simulink model "segway_ctrl_dt"  (R2020a)
settings: Solver=daessc  StartTime=0.0  StopTime=simlength  MaxStep=ts  RelTol=1e-3
values from neighbouring files (symbols this model uses):
  Ad = eye(4) + A*ts    [init_segway_ctrl.m]
  Aled = eye(5) + Ale*ts    [init_segway_ctrl.m]
  Bd = B*ts    [init_segway_ctrl.m]
  Bled = Ble*ts    [init_segway_ctrl.m]
  C = [1 0 0 0; 0 0 1 0]    [init_segway_ctrl.m]
  Cle = [1 0 0 0 0; 0 0 1 0 0]    [init_segway_ctrl.m]
  g = 9.8    [init_segway_ctrl.m]
  K1ed = (K1_hat+[0 0 0 0 1])/([Ad-eye(4) Bd; C1*Ad C1*Bd])    [init_segway_ctrl.m]
  K2ed = (K2_hat+[0 0 0 0 1])/([Ad-eye(4) Bd; C1*Ad C1*Bd])    [init_segway_ctrl.m]
  Ld = (place(Ad',C',poles_obsd))'    [init_segway_ctrl.m]
  Lled = (place(Aled',Cle',poles_obsd_le))'    [init_segway_ctrl.m]
  omega_1_ref = vref/r1    (= 28.5714285714)    [init_segway_ctrl.m]
  simlength = 20    [init_segway_ctrl.m]
  ts = 1e-3    (= 0.001)    [init_segway_ctrl.m]
libraries: nesl_utility x21, fl_lib x6, simulink x3, segway_lib x3
settings Model: SimulationMode=accelerator  Creator=dbagn  LastModifiedBy=dbagn
settings DataIOCC: ReturnWorkspaceOutputs=off

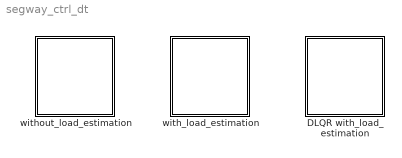
== system segway_ctrl_dt ==
  DLQR with_load_estimation : Subsystem
  with_load_estimation : Subsystem
  without_load_estimation : Subsystem

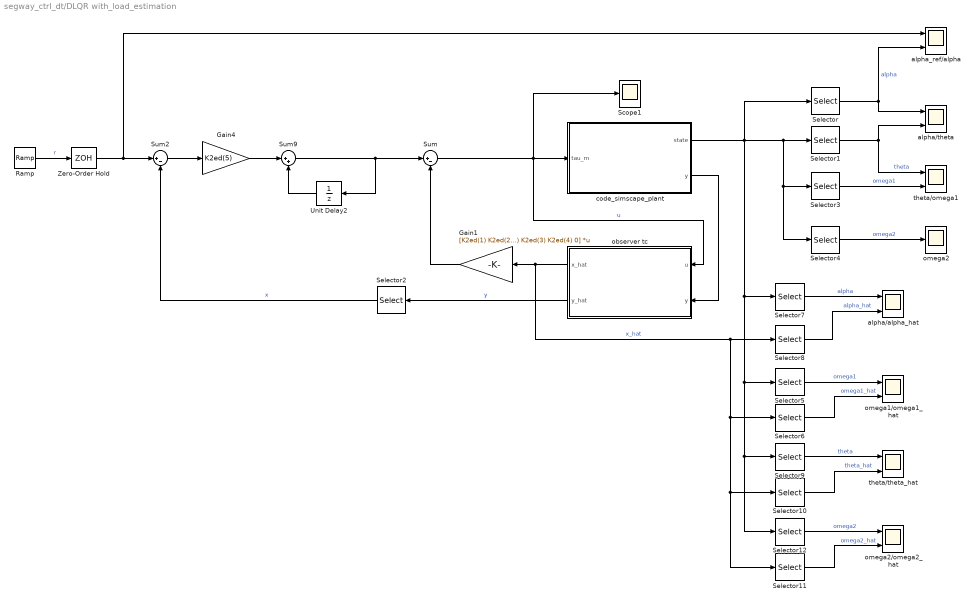
== system segway_ctrl_dt/DLQR with_load_estimation ==
  Gain1 : Gain  Gain=[K2ed(1) K2ed(2) K2ed(3) K2ed(4) 0]  Multiplication=Matrix(K*u)
  Gain4 : Gain  Gain=K2ed(5)
  Ramp : simulink/Sources/Ramp  slope=omega_1_ref  start=0  InitialOutput=0
  Scope1 : Scope
  Selector : Selector  InputPortWidth=4  IndexOptions=Index vector (dialog)  Indices=1  OutputSizes=1
  Selector1 : Selector  InputPortWidth=4  IndexOptions=Index vector (dialog)  Indices=3  OutputSizes=1
  Selector10 : Selector  InputPortWidth=5  IndexOptions=Index vector (dialog)  Indices=3  OutputSizes=1
  Selector11 : Selector  InputPortWidth=5  IndexOptions=Index vector (dialog)  Indices=4  OutputSizes=1
  Selector12 : Selector  InputPortWidth=4  IndexOptions=Index vector (dialog)  Indices=4  OutputSizes=1
  Selector2 : Selector  InputPortWidth=2  IndexOptions=Index vector (dialog)  Indices=1  OutputSizes=1
  Selector3 : Selector  InputPortWidth=4  IndexOptions=Index vector (dialog)  Indices=2  OutputSizes=1
  Selector4 : Selector  InputPortWidth=4  IndexOptions=Index vector (dialog)  Indices=4  OutputSizes=1
  Selector5 : Selector  InputPortWidth=4  IndexOptions=Index vector (dialog)  Indices=2  OutputSizes=1
  Selector6 : Selector  InputPortWidth=5  IndexOptions=Index vector (dialog)  Indices=2  OutputSizes=1
  Selector7 : Selector  InputPortWidth=4  IndexOptions=Index vector (dialog)  Indices=1  OutputSizes=1
  Selector8 : Selector  InputPortWidth=5  IndexOptions=Index vector (dialog)  Indices=1  OutputSizes=1
  Selector9 : Selector  InputPortWidth=4  IndexOptions=Index vector (dialog)  Indices=3  OutputSizes=1
  Sum : Sum  Inputs=|+-
  Sum2 : Sum  Inputs=|+-
  Sum9 : Sum  Inputs=|++
  Unit Delay2 : UnitDelay  SampleTime=ts  HasFrameUpgradeWarning=on
  Zero-Order Hold : ZeroOrderHold  SampleTime=ts
  alpha/alpha_hat : Scope  NumInputPorts=2
  alpha/theta : Scope  NumInputPorts=2
  alpha_ref/alpha : Scope  NumInputPorts=2
  "code_simscape_plant " : Subsystem
  observer tc : Subsystem
  omega1/omega1_hat : Scope  NumInputPorts=2
  omega2 : Scope
  omega2/omega2_hat : Scope  NumInputPorts=2
  theta/omega1 : Scope  NumInputPorts=2
  theta/theta_hat : Scope  NumInputPorts=2
  wires:
  Ramp/1 -> Zero-Order Hold/1  "r"
  Sum2/1 -> Gain4/1
  Gain4/1 -> Sum9/1
  Sum9/1 -> Unit Delay2/1, Sum/1
  Unit Delay2/1 -> Sum9/2
  Selector2/1 -> Sum2/2  "x"
  Zero-Order Hold/1 -> Sum2/1, alpha_ref/alpha/1
  Sum/1 -> Scope1/1, "code_simscape_plant "/1(tau_m), observer tc/1(u)  "u"
  Selector/1 -> alpha/theta/1, alpha_ref/alpha/2  "alpha"
  "code_simscape_plant "/1(state) -> Selector/1, Selector12/1, Selector9/1, Selector5/1, Selector7/1, Selector4/1, Selector3/1, Selector1/1
  "code_simscape_plant "/2(y) -> observer tc/2(y)
  Selector3/1 -> theta/omega1/2  "omega1"
  observer tc/1(x_hat) -> Selector8/1, Selector11/1, Selector10/1, Selector6/1, Gain1/1  "x_hat"
  Selector7/1 -> alpha/alpha_hat/1  "alpha"
  Selector1/1 -> theta/omega1/1, alpha/theta/2  "theta"
  Selector6/1 -> omega1/omega1_hat/2  "omega1_hat"
  Gain1/1 -> Sum/2
  observer tc/2(y_hat) -> Selector2/1  "y"
  Selector8/1 -> alpha/alpha_hat/2  "alpha_hat"
  Selector4/1 -> omega2/1  "omega2"
  Selector9/1 -> theta/theta_hat/1  "theta"
  Selector5/1 -> omega1/omega1_hat/1  "omega1"
  Selector10/1 -> theta/theta_hat/2  "theta_hat"
  Selector11/1 -> omega2/omega2_hat/2  "omega2_hat"
  Selector12/1 -> omega2/omega2_hat/1  "omega2"

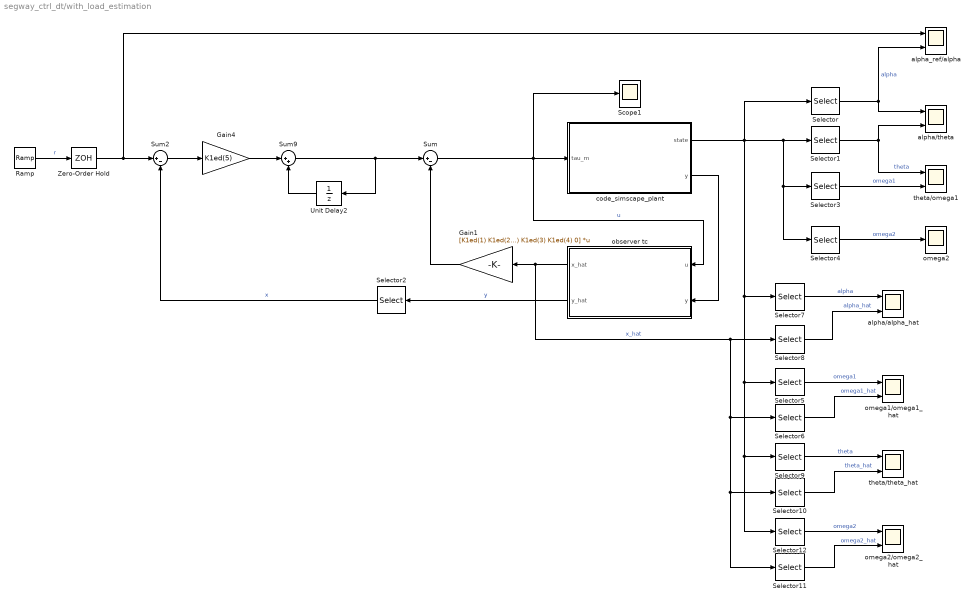
== system segway_ctrl_dt/with_load_estimation ==
  Gain1 : Gain  Gain=[K1ed(1) K1ed(2) K1ed(3) K1ed(4) 0]  Multiplication=Matrix(K*u)
  Gain4 : Gain  Gain=K1ed(5)
  Ramp : simulink/Sources/Ramp  slope=omega_1_ref  start=0  InitialOutput=0
  Scope1 : Scope
  Selector : Selector  InputPortWidth=4  IndexOptions=Index vector (dialog)  Indices=1  OutputSizes=1
  Selector1 : Selector  InputPortWidth=4  IndexOptions=Index vector (dialog)  Indices=3  OutputSizes=1
  Selector10 : Selector  InputPortWidth=5  IndexOptions=Index vector (dialog)  Indices=3  OutputSizes=1
  Selector11 : Selector  InputPortWidth=5  IndexOptions=Index vector (dialog)  Indices=4  OutputSizes=1
  Selector12 : Selector  InputPortWidth=4  IndexOptions=Index vector (dialog)  Indices=4  OutputSizes=1
  Selector2 : Selector  InputPortWidth=2  IndexOptions=Index vector (dialog)  Indices=1  OutputSizes=1
  Selector3 : Selector  InputPortWidth=4  IndexOptions=Index vector (dialog)  Indices=2  OutputSizes=1
  Selector4 : Selector  InputPortWidth=4  IndexOptions=Index vector (dialog)  Indices=4  OutputSizes=1
  Selector5 : Selector  InputPortWidth=4  IndexOptions=Index vector (dialog)  Indices=2  OutputSizes=1
  Selector6 : Selector  InputPortWidth=5  IndexOptions=Index vector (dialog)  Indices=2  OutputSizes=1
  Selector7 : Selector  InputPortWidth=4  IndexOptions=Index vector (dialog)  Indices=1  OutputSizes=1
  Selector8 : Selector  InputPortWidth=5  IndexOptions=Index vector (dialog)  Indices=1  OutputSizes=1
  Selector9 : Selector  InputPortWidth=4  IndexOptions=Index vector (dialog)  Indices=3  OutputSizes=1
  Sum : Sum  Inputs=|+-
  Sum2 : Sum  Inputs=|+-
  Sum9 : Sum  Inputs=|++
  Unit Delay2 : UnitDelay  SampleTime=ts  HasFrameUpgradeWarning=on
  Zero-Order Hold : ZeroOrderHold  SampleTime=ts
  alpha/alpha_hat : Scope  NumInputPorts=2
  alpha/theta : Scope  NumInputPorts=2
  alpha_ref/alpha : Scope  NumInputPorts=2
  "code_simscape_plant " : Subsystem
  observer tc : Subsystem
  omega1/omega1_hat : Scope  NumInputPorts=2
  omega2 : Scope
  omega2/omega2_hat : Scope  NumInputPorts=2
  theta/omega1 : Scope  NumInputPorts=2
  theta/theta_hat : Scope  NumInputPorts=2
  wires:
  Selector12/1 -> omega2/omega2_hat/1  "omega2"
  Selector11/1 -> omega2/omega2_hat/2  "omega2_hat"
  Selector10/1 -> theta/theta_hat/2  "theta_hat"
  Selector5/1 -> omega1/omega1_hat/1  "omega1"
  Selector9/1 -> theta/theta_hat/1  "theta"
  Selector4/1 -> omega2/1  "omega2"
  Selector8/1 -> alpha/alpha_hat/2  "alpha_hat"
  observer tc/2(y_hat) -> Selector2/1  "y"
  Gain1/1 -> Sum/2
  Selector6/1 -> omega1/omega1_hat/2  "omega1_hat"
  Selector1/1 -> alpha/theta/2, theta/omega1/1  "theta"
  Selector7/1 -> alpha/alpha_hat/1  "alpha"
  observer tc/1(x_hat) -> Gain1/1, Selector6/1, Selector10/1, Selector11/1, Selector8/1  "x_hat"
  Selector3/1 -> theta/omega1/2  "omega1"
  "code_simscape_plant "/2(y) -> observer tc/2(y)
  "code_simscape_plant "/1(state) -> Selector1/1, Selector3/1, Selector4/1, Selector7/1, Selector5/1, Selector9/1, Selector12/1, Selector/1
  Selector/1 -> alpha_ref/alpha/2, alpha/theta/1  "alpha"
  Sum/1 -> observer tc/1(u), "code_simscape_plant "/1(tau_m), Scope1/1  "u"
  Zero-Order Hold/1 -> alpha_ref/alpha/1, Sum2/1
  Selector2/1 -> Sum2/2  "x"
  Unit Delay2/1 -> Sum9/2
  Sum9/1 -> Sum/1, Unit Delay2/1
  Gain4/1 -> Sum9/1
  Sum2/1 -> Gain4/1
  Ramp/1 -> Zero-Order Hold/1  "r"

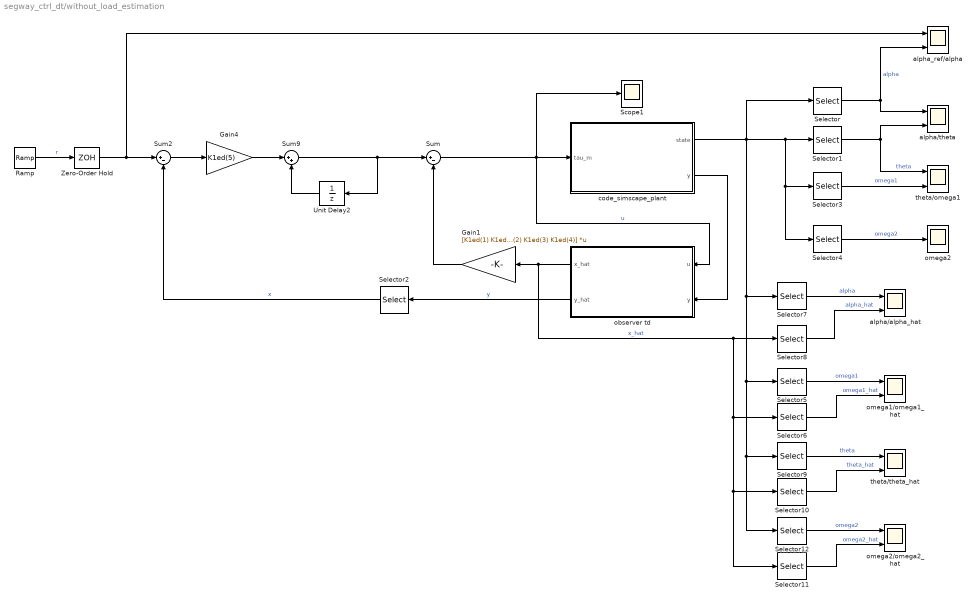
== system segway_ctrl_dt/without_load_estimation ==
  Gain1 : Gain  Gain=[K1ed(1) K1ed(2) K1ed(3) K1ed(4)]  Multiplication=Matrix(K*u)
  Gain4 : Gain  Gain=K1ed(5)
  Ramp : simulink/Sources/Ramp  slope=omega_1_ref  start=0  InitialOutput=0
  Scope1 : Scope
  Selector : Selector  InputPortWidth=4  IndexOptions=Index vector (dialog)  Indices=1  OutputSizes=1
  Selector1 : Selector  InputPortWidth=4  IndexOptions=Index vector (dialog)  Indices=3  OutputSizes=1
  Selector10 : Selector  InputPortWidth=4  IndexOptions=Index vector (dialog)  Indices=3  OutputSizes=1
  Selector11 : Selector  InputPortWidth=4  IndexOptions=Index vector (dialog)  Indices=4  OutputSizes=1
  Selector12 : Selector  InputPortWidth=4  IndexOptions=Index vector (dialog)  Indices=4  OutputSizes=1
  Selector2 : Selector  InputPortWidth=2  IndexOptions=Index vector (dialog)  Indices=1  OutputSizes=1
  Selector3 : Selector  InputPortWidth=4  IndexOptions=Index vector (dialog)  Indices=2  OutputSizes=1
  Selector4 : Selector  InputPortWidth=4  IndexOptions=Index vector (dialog)  Indices=4  OutputSizes=1
  Selector5 : Selector  InputPortWidth=4  IndexOptions=Index vector (dialog)  Indices=2  OutputSizes=1
  Selector6 : Selector  InputPortWidth=4  IndexOptions=Index vector (dialog)  Indices=2  OutputSizes=1
  Selector7 : Selector  InputPortWidth=4  IndexOptions=Index vector (dialog)  Indices=1  OutputSizes=1
  Selector8 : Selector  InputPortWidth=4  IndexOptions=Index vector (dialog)  Indices=1  OutputSizes=1
  Selector9 : Selector  InputPortWidth=4  IndexOptions=Index vector (dialog)  Indices=3  OutputSizes=1
  Sum : Sum  Inputs=|+-
  Sum2 : Sum  Inputs=|+-
  Sum9 : Sum  Inputs=|++
  Unit Delay2 : UnitDelay  SampleTime=ts  HasFrameUpgradeWarning=on
  Zero-Order Hold : ZeroOrderHold  SampleTime=ts
  alpha/alpha_hat : Scope  NumInputPorts=2
  alpha/theta : Scope  NumInputPorts=2
  alpha_ref/alpha : Scope  NumInputPorts=2
  "code_simscape_plant " : Subsystem
  observer td : Subsystem
  omega1/omega1_hat : Scope  NumInputPorts=2
  omega2 : Scope
  omega2/omega2_hat : Scope  NumInputPorts=2
  theta/omega1 : Scope  NumInputPorts=2
  theta/theta_hat : Scope  NumInputPorts=2
  wires:
  Sum/1 -> "code_simscape_plant "/1(tau_m), Scope1/1, observer td/1(u)  "u"
  Selector/1 -> alpha/theta/1, alpha_ref/alpha/2  "alpha"
  "code_simscape_plant "/1(state) -> Selector/1, Selector12/1, Selector9/1, Selector5/1, Selector7/1, Selector4/1, Selector3/1, Selector1/1
  "code_simscape_plant "/2(y) -> observer td/2(y)
  Selector3/1 -> theta/omega1/2  "omega1"
  observer td/1(x_hat) -> Selector8/1, Selector11/1, Selector10/1, Selector6/1, Gain1/1  "x_hat"
  Ramp/1 -> Zero-Order Hold/1  "r"
  Selector7/1 -> alpha/alpha_hat/1  "alpha"
  Selector1/1 -> theta/omega1/1, alpha/theta/2  "theta"
  Selector6/1 -> omega1/omega1_hat/2  "omega1_hat"
  Gain1/1 -> Sum/2
  Selector2/1 -> Sum2/2  "x"
  observer td/2(y_hat) -> Selector2/1  "y"
  Selector8/1 -> alpha/alpha_hat/2  "alpha_hat"
  Selector4/1 -> omega2/1  "omega2"
  Selector9/1 -> theta/theta_hat/1  "theta"
  Selector5/1 -> omega1/omega1_hat/1  "omega1"
  Selector10/1 -> theta/theta_hat/2  "theta_hat"
  Sum2/1 -> Gain4/1
  Selector11/1 -> omega2/omega2_hat/2  "omega2_hat"
  Selector12/1 -> omega2/omega2_hat/1  "omega2"
  Unit Delay2/1 -> Sum9/2
  Gain4/1 -> Sum9/1
  Sum9/1 -> Sum/1, Unit Delay2/1
  Zero-Order Hold/1 -> Sum2/1, alpha_ref/alpha/1

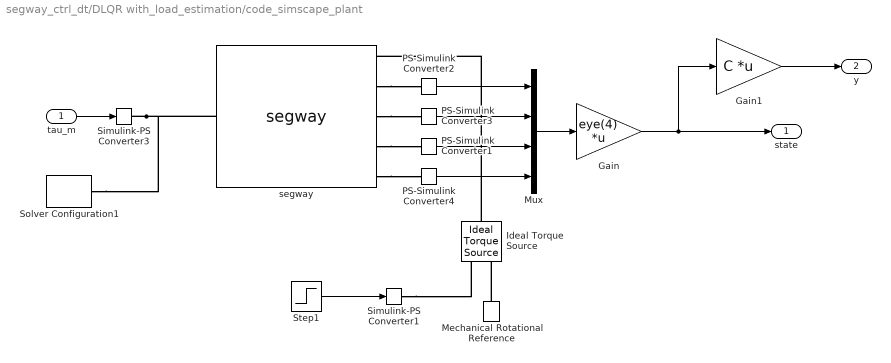
== system segway_ctrl_dt/DLQR with_load_estimation/code_simscape_plant  ==
  tau_m : Inport
  Gain : Gain  Gain=eye(4)  Multiplication=Matrix(K*u)
  Gain1 : Gain  Gain=C  Multiplication=Matrix(K*u)
  Ideal Torque Source : fl_lib/Mechanical/Mechanical Sources/Ideal Torque Source
  Mechanical Rotational Reference : fl_lib/Mechanical/Rotational Elements/Mechanical Rotational Reference
  Mux : Mux
  PS-Simulink Converter1 : nesl_utility/PS-Simulink Converter  PhysicalDomain=network_engine_domain  SubClassName=ps_output  LeftPortType=input  RightPortType=output  PseudoPeriodic=off  Frequencies=[]  Unit=rad  AffineConversion=on
  PS-Simulink Converter2 : nesl_utility/PS-Simulink Converter  PhysicalDomain=network_engine_domain  SubClassName=ps_output  LeftPortType=input  RightPortType=output  PseudoPeriodic=off  Frequencies=[]  Unit=rad  AffineConversion=on
  PS-Simulink Converter3 : nesl_utility/PS-Simulink Converter  PhysicalDomain=network_engine_domain  SubClassName=ps_output  LeftPortType=input  RightPortType=output  PseudoPeriodic=off  Frequencies=[]  Unit=rad/s  AffineConversion=on
  PS-Simulink Converter4 : nesl_utility/PS-Simulink Converter  PhysicalDomain=network_engine_domain  SubClassName=ps_output  LeftPortType=input  RightPortType=output  PseudoPeriodic=off  Frequencies=[]  Unit=rad/s  AffineConversion=on
  Simulink-PS Converter1 : nesl_utility/Simulink-PS Converter  PhysicalDomain=network_engine_domain  SubClassName=ps_input  LeftPortType=input  RightPortType=output  PseudoPeriodic=off  Frequencies=[]  NoiseDistribution=none  NoiseParameters=[]  Unit=N*m  AffineConversion=off  FilteringAndDerivatives=provide  SimscapeFilterOrder=1  InputFilterTimeConstant=0.001  UdotUserProvided=0
  Simulink-PS Converter3 : nesl_utility/Simulink-PS Converter  PhysicalDomain=network_engine_domain  SubClassName=ps_input  LeftPortType=input  RightPortType=output  PseudoPeriodic=off  Frequencies=[]  NoiseDistribution=none  NoiseParameters=[]  Unit=N*m  AffineConversion=off  FilteringAndDerivatives=provide  SimscapeFilterOrder=1  InputFilterTimeConstant=0.001  UdotUserProvided=0
  Solver Configuration1 : nesl_utility/Solver Configuration  PhysicalDomain=network_engine_domain  SubClassName=solver  LeftPortType=input  RightPortType=generic  Tones=[]  Harmonics=[]  SimulateNoise=off  Profile=off  UseLocalSampling=off  EnableSwitchedLinearOptims=on  FrequencyDomain=off  UseCCode=off  RelTol=0.001  AbsTol=1e-06  MinStep=1e-09  ToWorkspace=off  RevertToSquareIcSolve=off  NumHomotopyIterations=100  PhasorMode=off  PhasorModeNumHarmonics=1  DoDC=on  ResidualTolerance=1e-09  UseLocalSolver=on  LocalSolverChoice=NE_BACKWARD_EULER_ADVANCER  LocalSolverSampleTime=ts  DoFixedCost=on  MaxNonlinIter=3  MaxModeIter=2  LinearAlgebra=auto  EquationFormulation=NE_TIME_EF  DelaysMemoryBudget=1024  AutomaticFiltering=on  FilteringTimeConstant=0.001  PartitionStorageMethod=AS_NEEDED  PartitionMemoryBudget=1024  PartitionMethod=ROBUST
  Step1 : Step  Time=simlength/2  After=250  SampleTime=0
  segway : segway_lib/segway  m1=m1 kg  m2=m2 kg  J1=J1 kg*m^2  J2=J2 kg*m^2  r1=r1 m  r2=r2 m  b1=b1 N*m/(rad/s)  b2=b2 N*m/(rad/s)  g=g m/s^2  d_specify=off  d_priority=None  d=0 N*m  d_nominal_specify=off  d_nominal_unit=N*m  d_nominal_value=1  x1_specify=off  x1_priority=None  x1=0 rad  x1_nominal_specify=off  x1_nominal_unit=rad  x1_nominal_value=1  x2_specify=off  x2_priority=None  x2=0 rad/s  x2_nominal_specify=off  x2_nominal_unit=rad/s  x2_nominal_value=1  x3_specify=on  x3_priority=High  x3=1 rad  x3_nominal_specify=off  x3_nominal_unit=rad  x3_nominal_value=1  x4_specify=on  x4_priority=High  x4=0 rad/s  x4_nominal_specify=off  x4_nominal_unit=rad/s  x4_nominal_value=1
      settings: InternalSimscapePortConfiguration="{\"Bottom\":[],\"Left\":[{\"id\":\"tau_m\",\"label\":\"tau_m\",\"type\":\"input\"}],\"Right\":[{\"id\":\"S1\",\"label\":\"S1\",\"type\":\"foundation.mechanical.rotational.rotational\"},{\"id\":\"alpha\",\"label\":\"alpha\",\"type\":\"output\"},{\"id\":\"omega_1\",\"label\":\"omega_1\",\"type\":\"output\"},{\"id\":\"theta\",\"label\":\"theta\",\"type\":\"output\"},{\"id\":\"omega_2\",\"label\":\"omega_2\",\"type\":\"output\"}],\"Top\":[]}"
  state : Outport
  y : Outport  Port=2
  wires:
  PS-Simulink Converter2/1 -> Mux/1
  PS-Simulink Converter3/1 -> Mux/2
  tau_m/1 -> Simulink-PS Converter3/1
  PS-Simulink Converter1/1 -> Mux/3
  PS-Simulink Converter4/1 -> Mux/4
  Mux/1 -> Gain/1
  Gain/1 -> Gain1/1, state/1
  Gain1/1 -> y/1
  Step1/1 -> Simulink-PS Converter1/1
  connections:
  Simulink-PS Converter1/RConn1 -- Ideal Torque Source/RConn1
  Ideal Torque Source/LConn1 -- segway/RConn1
  Mechanical Rotational Reference/LConn1 -- Ideal Torque Source/RConn2
  segway/RConn5 -- PS-Simulink Converter4/LConn1
  segway/RConn4 -- PS-Simulink Converter1/LConn1
  segway/RConn3 -- PS-Simulink Converter3/LConn1
  segway/RConn2 -- PS-Simulink Converter2/LConn1
  Simulink-PS Converter3/RConn1 -- Solver Configuration1/RConn1 -- segway/LConn1

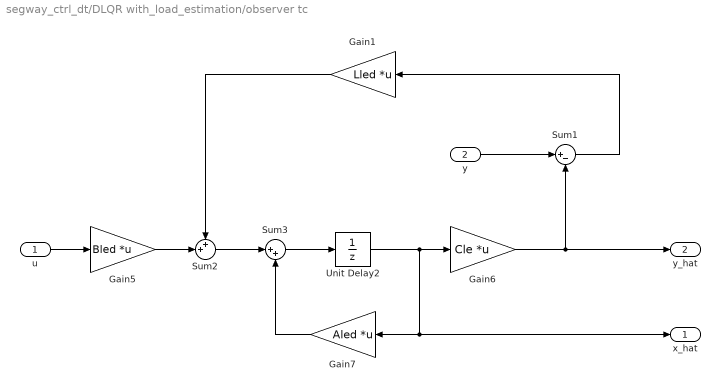
== system segway_ctrl_dt/DLQR with_load_estimation/observer tc ==
  u : Inport
  y : Inport  Port=2
  Gain1 : Gain  Gain=Lled  Multiplication=Matrix(K*u)
  Gain5 : Gain  Gain=Bled  Multiplication=Matrix(K*u)
  Gain6 : Gain  Gain=Cle  Multiplication=Matrix(K*u)
  Gain7 : Gain  Gain=Aled  Multiplication=Matrix(K*u)
  Sum1 : Sum  Inputs=|+-
  Sum2 : Sum  Inputs=++|
  Sum3 : Sum  Inputs=|++
  Unit Delay2 : UnitDelay  SampleTime=ts  HasFrameUpgradeWarning=on
  x_hat : Outport
  y_hat : Outport  Port=2
  wires:
  Unit Delay2/1 -> x_hat/1, Gain7/1, Gain6/1
  Sum2/1 -> Sum3/1
  Sum3/1 -> Unit Delay2/1
  Gain7/1 -> Sum3/2
  y/1 -> Sum1/1
  Gain6/1 -> y_hat/1, Sum1/2
  Sum1/1 -> Gain1/1
  u/1 -> Gain5/1
  Gain1/1 -> Sum2/1
  Gain5/1 -> Sum2/2

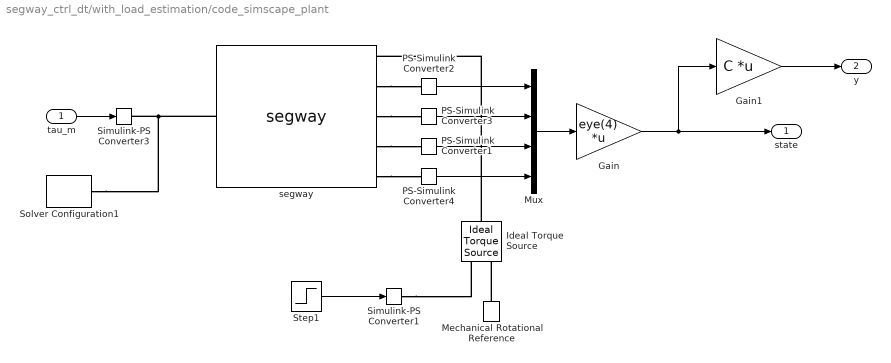
== system segway_ctrl_dt/with_load_estimation/code_simscape_plant  ==
  tau_m : Inport
  Gain : Gain  Gain=eye(4)  Multiplication=Matrix(K*u)
  Gain1 : Gain  Gain=C  Multiplication=Matrix(K*u)
  Ideal Torque Source : fl_lib/Mechanical/Mechanical Sources/Ideal Torque Source
  Mechanical Rotational Reference : fl_lib/Mechanical/Rotational Elements/Mechanical Rotational Reference
  Mux : Mux
  PS-Simulink Converter1 : nesl_utility/PS-Simulink Converter  PhysicalDomain=network_engine_domain  SubClassName=ps_output  LeftPortType=input  RightPortType=output  PseudoPeriodic=off  Frequencies=[]  Unit=rad  AffineConversion=on
  PS-Simulink Converter2 : nesl_utility/PS-Simulink Converter  PhysicalDomain=network_engine_domain  SubClassName=ps_output  LeftPortType=input  RightPortType=output  PseudoPeriodic=off  Frequencies=[]  Unit=rad  AffineConversion=on
  PS-Simulink Converter3 : nesl_utility/PS-Simulink Converter  PhysicalDomain=network_engine_domain  SubClassName=ps_output  LeftPortType=input  RightPortType=output  PseudoPeriodic=off  Frequencies=[]  Unit=rad/s  AffineConversion=on
  PS-Simulink Converter4 : nesl_utility/PS-Simulink Converter  PhysicalDomain=network_engine_domain  SubClassName=ps_output  LeftPortType=input  RightPortType=output  PseudoPeriodic=off  Frequencies=[]  Unit=rad/s  AffineConversion=on
  Simulink-PS Converter1 : nesl_utility/Simulink-PS Converter  PhysicalDomain=network_engine_domain  SubClassName=ps_input  LeftPortType=input  RightPortType=output  PseudoPeriodic=off  Frequencies=[]  NoiseDistribution=none  NoiseParameters=[]  Unit=N*m  AffineConversion=off  FilteringAndDerivatives=provide  SimscapeFilterOrder=1  InputFilterTimeConstant=0.001  UdotUserProvided=0
  Simulink-PS Converter3 : nesl_utility/Simulink-PS Converter  PhysicalDomain=network_engine_domain  SubClassName=ps_input  LeftPortType=input  RightPortType=output  PseudoPeriodic=off  Frequencies=[]  NoiseDistribution=none  NoiseParameters=[]  Unit=N*m  AffineConversion=off  FilteringAndDerivatives=provide  SimscapeFilterOrder=1  InputFilterTimeConstant=0.001  UdotUserProvided=0
  Solver Configuration1 : nesl_utility/Solver Configuration  PhysicalDomain=network_engine_domain  SubClassName=solver  LeftPortType=input  RightPortType=generic  Tones=[]  Harmonics=[]  SimulateNoise=off  Profile=off  UseLocalSampling=off  EnableSwitchedLinearOptims=on  FrequencyDomain=off  UseCCode=off  RelTol=0.001  AbsTol=1e-06  MinStep=1e-09  ToWorkspace=off  RevertToSquareIcSolve=off  NumHomotopyIterations=100  PhasorMode=off  PhasorModeNumHarmonics=1  DoDC=on  ResidualTolerance=1e-09  UseLocalSolver=on  LocalSolverChoice=NE_BACKWARD_EULER_ADVANCER  LocalSolverSampleTime=ts  DoFixedCost=on  MaxNonlinIter=3  MaxModeIter=2  LinearAlgebra=auto  EquationFormulation=NE_TIME_EF  DelaysMemoryBudget=1024  AutomaticFiltering=on  FilteringTimeConstant=0.001  PartitionStorageMethod=AS_NEEDED  PartitionMemoryBudget=1024  PartitionMethod=ROBUST
  Step1 : Step  Time=simlength/2  After=250  SampleTime=0
  segway : segway_lib/segway  m1=m1 kg  m2=m2 kg  J1=J1 kg*m^2  J2=J2 kg*m^2  r1=r1 m  r2=r2 m  b1=b1 N*m/(rad/s)  b2=b2 N*m/(rad/s)  g=g m/s^2  d_specify=off  d_priority=None  d=0 N*m  d_nominal_specify=off  d_nominal_unit=N*m  d_nominal_value=1  x1_specify=off  x1_priority=None  x1=0 rad  x1_nominal_specify=off  x1_nominal_unit=rad  x1_nominal_value=1  x2_specify=off  x2_priority=None  x2=0 rad/s  x2_nominal_specify=off  x2_nominal_unit=rad/s  x2_nominal_value=1  x3_specify=on  x3_priority=High  x3=1 rad  x3_nominal_specify=off  x3_nominal_unit=rad  x3_nominal_value=1  x4_specify=on  x4_priority=High  x4=0 rad/s  x4_nominal_specify=off  x4_nominal_unit=rad/s  x4_nominal_value=1
      settings: InternalSimscapePortConfiguration="{\"Bottom\":[],\"Left\":[{\"id\":\"tau_m\",\"label\":\"tau_m\",\"type\":\"input\"}],\"Right\":[{\"id\":\"S1\",\"label\":\"S1\",\"type\":\"foundation.mechanical.rotational.rotational\"},{\"id\":\"alpha\",\"label\":\"alpha\",\"type\":\"output\"},{\"id\":\"omega_1\",\"label\":\"omega_1\",\"type\":\"output\"},{\"id\":\"theta\",\"label\":\"theta\",\"type\":\"output\"},{\"id\":\"omega_2\",\"label\":\"omega_2\",\"type\":\"output\"}],\"Top\":[]}"
  state : Outport
  y : Outport  Port=2
  wires:
  Step1/1 -> Simulink-PS Converter1/1
  Gain1/1 -> y/1
  Gain/1 -> state/1, Gain1/1
  Mux/1 -> Gain/1
  PS-Simulink Converter4/1 -> Mux/4
  PS-Simulink Converter1/1 -> Mux/3
  tau_m/1 -> Simulink-PS Converter3/1
  PS-Simulink Converter3/1 -> Mux/2
  PS-Simulink Converter2/1 -> Mux/1
  connections:
  segway/LConn1 -- Solver Configuration1/RConn1 -- Simulink-PS Converter3/RConn1
  segway/RConn2 -- PS-Simulink Converter2/LConn1
  segway/RConn3 -- PS-Simulink Converter3/LConn1
  segway/RConn4 -- PS-Simulink Converter1/LConn1
  segway/RConn5 -- PS-Simulink Converter4/LConn1
  Mechanical Rotational Reference/LConn1 -- Ideal Torque Source/RConn2
  Ideal Torque Source/LConn1 -- segway/RConn1
  Simulink-PS Converter1/RConn1 -- Ideal Torque Source/RConn1

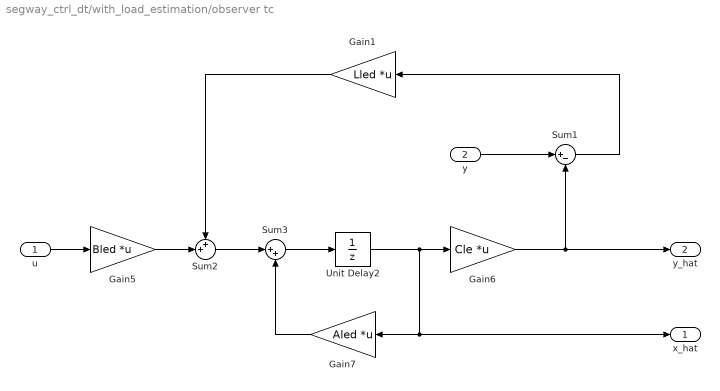
== system segway_ctrl_dt/with_load_estimation/observer tc ==
  u : Inport
  y : Inport  Port=2
  Gain1 : Gain  Gain=Lled  Multiplication=Matrix(K*u)
  Gain5 : Gain  Gain=Bled  Multiplication=Matrix(K*u)
  Gain6 : Gain  Gain=Cle  Multiplication=Matrix(K*u)
  Gain7 : Gain  Gain=Aled  Multiplication=Matrix(K*u)
  Sum1 : Sum  Inputs=|+-
  Sum2 : Sum  Inputs=++|
  Sum3 : Sum  Inputs=|++
  Unit Delay2 : UnitDelay  SampleTime=ts  HasFrameUpgradeWarning=on
  x_hat : Outport
  y_hat : Outport  Port=2
  wires:
  Gain5/1 -> Sum2/2
  Gain1/1 -> Sum2/1
  u/1 -> Gain5/1
  Sum1/1 -> Gain1/1
  Gain6/1 -> Sum1/2, y_hat/1
  y/1 -> Sum1/1
  Gain7/1 -> Sum3/2
  Sum3/1 -> Unit Delay2/1
  Sum2/1 -> Sum3/1
  Unit Delay2/1 -> Gain6/1, Gain7/1, x_hat/1

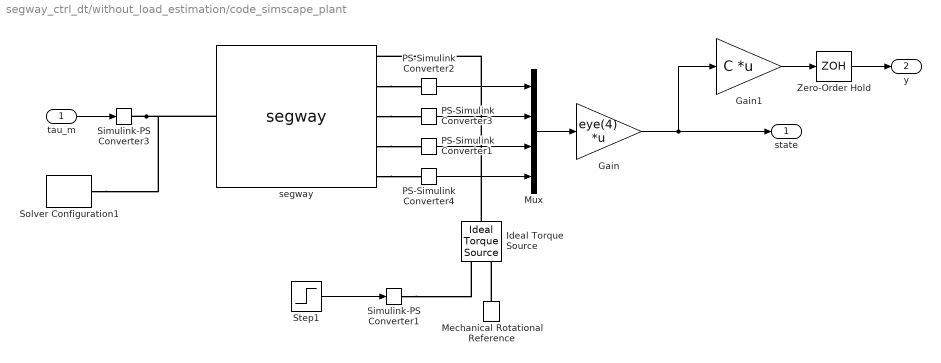
== system segway_ctrl_dt/without_load_estimation/code_simscape_plant  ==
  tau_m : Inport
  Gain : Gain  Gain=eye(4)  Multiplication=Matrix(K*u)
  Gain1 : Gain  Gain=C  Multiplication=Matrix(K*u)
  Ideal Torque Source : fl_lib/Mechanical/Mechanical Sources/Ideal Torque Source
  Mechanical Rotational Reference : fl_lib/Mechanical/Rotational Elements/Mechanical Rotational Reference
  Mux : Mux
  PS-Simulink Converter1 : nesl_utility/PS-Simulink Converter  PhysicalDomain=network_engine_domain  SubClassName=ps_output  LeftPortType=input  RightPortType=output  PseudoPeriodic=off  Frequencies=[]  Unit=rad  AffineConversion=on
  PS-Simulink Converter2 : nesl_utility/PS-Simulink Converter  PhysicalDomain=network_engine_domain  SubClassName=ps_output  LeftPortType=input  RightPortType=output  PseudoPeriodic=off  Frequencies=[]  Unit=rad  AffineConversion=on
  PS-Simulink Converter3 : nesl_utility/PS-Simulink Converter  PhysicalDomain=network_engine_domain  SubClassName=ps_output  LeftPortType=input  RightPortType=output  PseudoPeriodic=off  Frequencies=[]  Unit=rad/s  AffineConversion=on
  PS-Simulink Converter4 : nesl_utility/PS-Simulink Converter  PhysicalDomain=network_engine_domain  SubClassName=ps_output  LeftPortType=input  RightPortType=output  PseudoPeriodic=off  Frequencies=[]  Unit=rad/s  AffineConversion=on
  Simulink-PS Converter1 : nesl_utility/Simulink-PS Converter  PhysicalDomain=network_engine_domain  SubClassName=ps_input  LeftPortType=input  RightPortType=output  PseudoPeriodic=off  Frequencies=[]  NoiseDistribution=none  NoiseParameters=[]  Unit=N*m  AffineConversion=off  FilteringAndDerivatives=provide  SimscapeFilterOrder=1  InputFilterTimeConstant=0.001  UdotUserProvided=0
  Simulink-PS Converter3 : nesl_utility/Simulink-PS Converter  PhysicalDomain=network_engine_domain  SubClassName=ps_input  LeftPortType=input  RightPortType=output  PseudoPeriodic=off  Frequencies=[]  NoiseDistribution=none  NoiseParameters=[]  Unit=N*m  AffineConversion=off  FilteringAndDerivatives=provide  SimscapeFilterOrder=1  InputFilterTimeConstant=0.001  UdotUserProvided=0
  Solver Configuration1 : nesl_utility/Solver Configuration  PhysicalDomain=network_engine_domain  SubClassName=solver  LeftPortType=input  RightPortType=generic  Tones=[]  Harmonics=[]  SimulateNoise=off  Profile=off  UseLocalSampling=off  EnableSwitchedLinearOptims=on  FrequencyDomain=off  UseCCode=off  RelTol=0.001  AbsTol=1e-06  MinStep=1e-09  ToWorkspace=off  RevertToSquareIcSolve=off  NumHomotopyIterations=100  PhasorMode=off  PhasorModeNumHarmonics=1  DoDC=on  ResidualTolerance=1e-09  UseLocalSolver=on  LocalSolverChoice=NE_BACKWARD_EULER_ADVANCER  LocalSolverSampleTime=ts  DoFixedCost=on  MaxNonlinIter=3  MaxModeIter=2  LinearAlgebra=auto  EquationFormulation=NE_TIME_EF  DelaysMemoryBudget=1024  AutomaticFiltering=on  FilteringTimeConstant=0.001  PartitionStorageMethod=AS_NEEDED  PartitionMemoryBudget=1024  PartitionMethod=ROBUST
  Step1 : Step  Time=simlength/2  After=250  SampleTime=0
  Zero-Order Hold : ZeroOrderHold  SampleTime=ts
  segway : segway_lib/segway  m1=m1 kg  m2=m2 kg  J1=J1 kg*m^2  J2=J2 kg*m^2  r1=r1 m  r2=r2 m  b1=b1 N*m/(rad/s)  b2=b2 N*m/(rad/s)  g=g m/s^2  d_specify=off  d_priority=None  d=0 N*m  d_nominal_specify=off  d_nominal_unit=N*m  d_nominal_value=1  x1_specify=off  x1_priority=None  x1=0 rad  x1_nominal_specify=off  x1_nominal_unit=rad  x1_nominal_value=1  x2_specify=off  x2_priority=None  x2=0 rad/s  x2_nominal_specify=off  x2_nominal_unit=rad/s  x2_nominal_value=1  x3_specify=on  x3_priority=High  x3=1 rad  x3_nominal_specify=off  x3_nominal_unit=rad  x3_nominal_value=1  x4_specify=on  x4_priority=High  x4=0 rad/s  x4_nominal_specify=off  x4_nominal_unit=rad/s  x4_nominal_value=1
      settings: InternalSimscapePortConfiguration="{\"Bottom\":[],\"Left\":[{\"id\":\"tau_m\",\"label\":\"tau_m\",\"type\":\"input\"}],\"Right\":[{\"id\":\"S1\",\"label\":\"S1\",\"type\":\"foundation.mechanical.rotational.rotational\"},{\"id\":\"alpha\",\"label\":\"alpha\",\"type\":\"output\"},{\"id\":\"omega_1\",\"label\":\"omega_1\",\"type\":\"output\"},{\"id\":\"theta\",\"label\":\"theta\",\"type\":\"output\"},{\"id\":\"omega_2\",\"label\":\"omega_2\",\"type\":\"output\"}],\"Top\":[]}"
  state : Outport
  y : Outport  Port=2
  wires:
  Step1/1 -> Simulink-PS Converter1/1
  Gain1/1 -> Zero-Order Hold/1
  Gain/1 -> state/1, Gain1/1
  Mux/1 -> Gain/1
  PS-Simulink Converter4/1 -> Mux/4
  PS-Simulink Converter1/1 -> Mux/3
  tau_m/1 -> Simulink-PS Converter3/1
  PS-Simulink Converter3/1 -> Mux/2
  PS-Simulink Converter2/1 -> Mux/1
  Zero-Order Hold/1 -> y/1
  connections:
  Simulink-PS Converter3/RConn1 -- segway/LConn1 -- Solver Configuration1/RConn1
  segway/RConn2 -- PS-Simulink Converter2/LConn1
  segway/RConn3 -- PS-Simulink Converter3/LConn1
  segway/RConn4 -- PS-Simulink Converter1/LConn1
  segway/RConn5 -- PS-Simulink Converter4/LConn1
  Mechanical Rotational Reference/LConn1 -- Ideal Torque Source/RConn2
  Ideal Torque Source/LConn1 -- segway/RConn1
  Simulink-PS Converter1/RConn1 -- Ideal Torque Source/RConn1

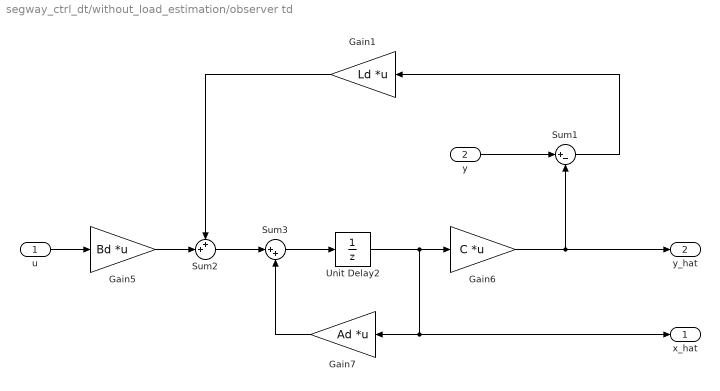
== system segway_ctrl_dt/without_load_estimation/observer td ==
  u : Inport
  y : Inport  Port=2
  Gain1 : Gain  Gain=Ld  Multiplication=Matrix(K*u)
  Gain5 : Gain  Gain=Bd  Multiplication=Matrix(K*u)
  Gain6 : Gain  Gain=C  Multiplication=Matrix(K*u)
  Gain7 : Gain  Gain=Ad  Multiplication=Matrix(K*u)
  Sum1 : Sum  Inputs=|+-
  Sum2 : Sum  Inputs=++|
  Sum3 : Sum  Inputs=|++
  Unit Delay2 : UnitDelay  SampleTime=ts  HasFrameUpgradeWarning=on
  x_hat : Outport
  y_hat : Outport  Port=2
  wires:
  Sum2/1 -> Sum3/1
  Sum3/1 -> Unit Delay2/1
  Gain7/1 -> Sum3/2
  y/1 -> Sum1/1
  Gain6/1 -> y_hat/1, Sum1/2
  Sum1/1 -> Gain1/1
  u/1 -> Gain5/1
  Gain1/1 -> Sum2/1
  Gain5/1 -> Sum2/2
  Unit Delay2/1 -> x_hat/1, Gain7/1, Gain6/1
